simulink model "update_flight_mode"  (R2016a)
settings: Solver=VariableStepAuto  StartTime=0.0  StopTime=10.0  RelTol=1e-3
settings Model: Creator=GusBus  LastModifiedBy=GusBus
settings GRTTargetCC: GeneratePreprocessorConditionals=Use local settings

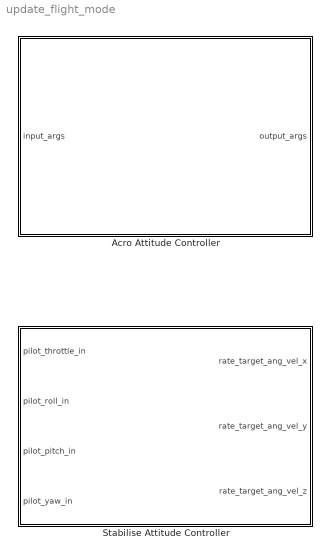
== system update_flight_mode ==
  Acro Attitude Controller : MATLAB Function  TreatAsAtomicUnit=on
  Stabilise Attitude Controller : MATLAB Function  TreatAsAtomicUnit=on

== matlab function update_flight_mode/Acro Attitude Controller ==
  data: input_args input; output_args output
function output_args   = acro_run( input_args )
%% acro_run
    
    
end

== matlab function update_flight_mode/Stabilise Attitude Controller ==
  data: pilot_throttle_in input; rate_target_ang_vel_x output; pilot_roll_in input; pilot_pitch_in input; pilot_yaw_in input; rate_target_ang_vel_y output; rate_target_ang_vel_z output
function [rate_target_ang_vel_x, rate_target_ang_vel_y, rate_target_ang_vel_z]   = stabilise_run( pilot_throttle_in, pilot_roll_in, pilot_pitch_in, pilot_yaw_in)
%% stabilise_run
%
% void Copter::stabilize_run()
% {
%     float target_roll, target_pitch;
%     float target_yaw_rate;
%     float pilot_throttle_scaled;
% 
%     // convert pilot input to lean angles
%     // To-Do: convert get_pilot_desired_lean_angles to return angles as floats
%     get_pilot_desired_lean_angles(channel_roll->get_control_in(), channel_pitch->get_control_in(), target_roll, target_pitch, aparm.angle_max);
% 
%     // get pilot's desired yaw rate
%     target_yaw_rate = get_pilot_desired_yaw_rate(channel_yaw->get_control_in());
% 
%     // get pilot's desired throttle
%     pilot_throttle_scaled = get_pilot_desired_throttle(channel_throttle->get_control_in());
% 
%     // call attitude controller
%     attitude_control.input_euler_angle_roll_pitch_euler_rate_yaw(target_roll, target_pitch, target_yaw_rate, get_smoothing_gain());
% 
%     // body-frame rate controller is run directly from 100hz loop
% 
%     // output pilot's throttle
%     attitude_control.set_throttle_out(pilot_throttle_scaled, true, g.throttle_filt);
% }
    %% Declare Global Variables
    global throttle_in throttle_avg_max
    
    %% Declare Function Variables
    float target_roll target_pitch
    float target_yaw_rate
    float pilot_throttle_scaled
    
    %% Scale Pilot Inputs
    [target_roll, target_pitch] = get_pilot_desired_lean_angles(pilot_roll_in, pilot_pitch_in, aparm.angle_max);
    target_yaw_rate = get_pilot_desired_yaw_rate(pilot_yaw_in);
    pilot_throttle_scaled = get_pilot_desired_throttle(pilot_throttle_in);
    
    %% Run the Attitude Controller
    [rate_target_ang_vel_x, rate_target_ang_vel_y, rate_target_ang_vel_z] = input_euler_angle_roll_pitch_euler_rate_yaw(target_roll, target_pitch, target_yaw_rate, get_smoothing_gain());
    [throttle_in, throttle_avg_max] = set_throttle_out(pilot_throttle_scaled);
    
end
